simulink model "TurbochargerFullMap"  (R2014b)
settings: Solver=ode45  StartTime=0.0  StopTime=10.0  RelTol=1e-3
undefined symbols (not defined in the file or in its folder): eng
settings Model: Creator=yum  LastModifiedBy=yum

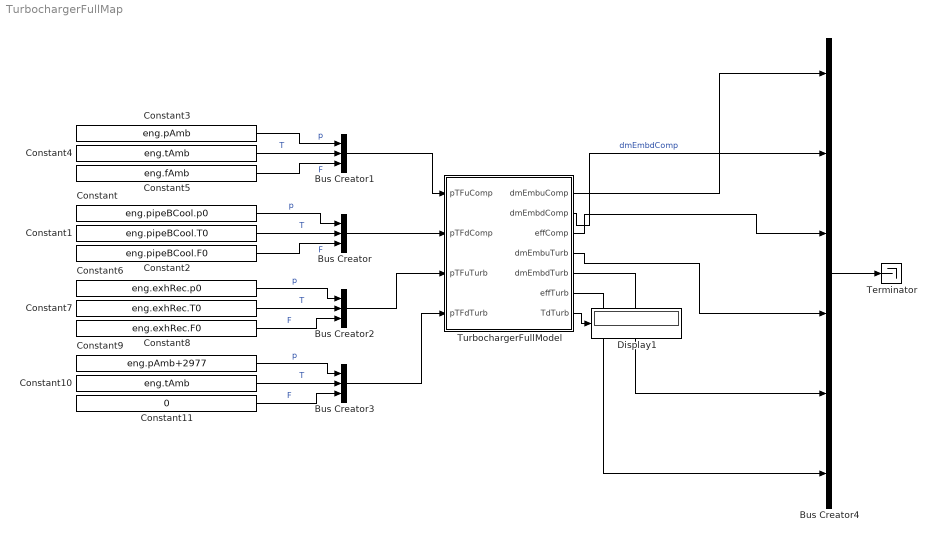
== system TurbochargerFullMap ==
  Bus Creator{,1..3} (4 alike) : BusCreator  Inputs=3
  Bus Creator4 : BusCreator  Inputs=6
  Constant : Constant  Value=eng.pipeBCool.p0
  Constant1 : Constant  Value=eng.pipeBCool.T0
  Constant10 : Constant  Value=eng.tAmb
  Constant11 : Constant  Value=0
  Constant2 : Constant  Value=eng.pipeBCool.F0
  Constant3 : Constant  Value=eng.pAmb
  Constant4 : Constant  Value=eng.tAmb
  Constant5 : Constant  Value=eng.fAmb
  Constant6 : Constant  Value=eng.exhRec.p0
  Constant7 : Constant  Value=eng.exhRec.T0
  Constant8 : Constant  Value=eng.exhRec.F0
  Constant9 : Constant  Value=eng.pAmb+2977
  Display1 : Display
  Terminator : Terminator
  TurbochargerFullModel : Subsystem  mask{turbo=eng.turbo}
      mask prompts: turbo "Turbocharger parameters"
  wires:
  Bus Creator/1 -> TurbochargerFullModel/2(pTFdComp)
  Constant/1 -> Bus Creator/1  "p"
  Constant1/1 -> Bus Creator/2  "T"
  Constant2/1 -> Bus Creator/3  "F"
  Constant4/1 -> Bus Creator1/2  "T"
  Constant5/1 -> Bus Creator1/3  "F"
  Constant3/1 -> Bus Creator1/1  "p"
  Bus Creator1/1 -> TurbochargerFullModel/1(pTFuComp)
  Constant6/1 -> Bus Creator2/1  "p"
  Constant7/1 -> Bus Creator2/2  "T"
  Constant8/1 -> Bus Creator2/3  "F"
  Bus Creator2/1 -> TurbochargerFullModel/3(pTFuTurb)
  Constant9/1 -> Bus Creator3/1  "p"
  Constant10/1 -> Bus Creator3/2  "T"
  Constant11/1 -> Bus Creator3/3  "F"
  Bus Creator3/1 -> TurbochargerFullModel/4(pTFdTurb)
  Bus Creator4/1 -> Terminator/1
  TurbochargerFullModel/3(effComp) -> Bus Creator4/3
  TurbochargerFullModel/4(dmEmbuTurb) -> Bus Creator4/4
  TurbochargerFullModel/2(dmEmbdComp) -> Bus Creator4/2  "dmEmbdComp"
  TurbochargerFullModel/5(dmEmbdTurb) -> Bus Creator4/5
  TurbochargerFullModel/1(dmEmbuComp) -> Bus Creator4/1
  TurbochargerFullModel/6(effTurb) -> Bus Creator4/6
  TurbochargerFullModel/7(TdTurb) -> Display1/1

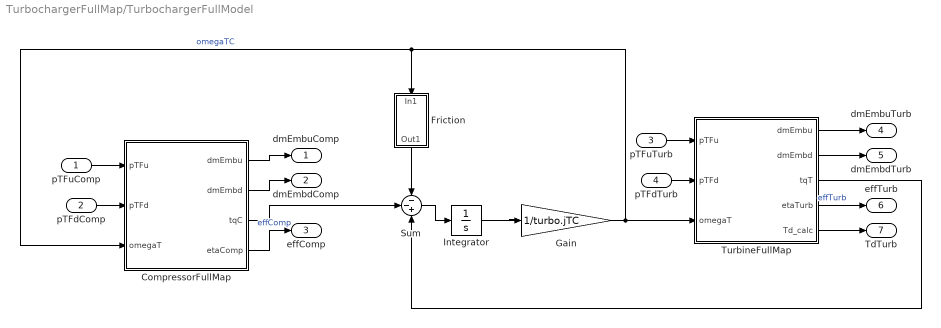
== system TurbochargerFullMap/TurbochargerFullModel ==
  pTFuComp : Inport
  pTFdComp : Inport  Port=2
  pTFuTurb : Inport  Port=3
  pTFdTurb : Inport  Port=4
  CompressorFullMap : Subsystem  mask{comp=turbo.comp}
      mask prompts: comp "Compressor Parameters"
  Friction : Subsystem
  Gain : Gain  Gain=1/turbo.jTC
  Integrator : Integrator  InitialCondition=turbo.jTC*1200
  Sum : Sum  Inputs=--+
  TurbineFullMap : Subsystem  mask{turb=turbo.turb}
      mask prompts: turb "Turbine parameters"
  dmEmbuComp : Outport
  dmEmbdComp : Outport  Port=2
  effComp : Outport  Port=3
  dmEmbuTurb : Outport  Port=4
  dmEmbdTurb : Outport  Port=5
  effTurb : Outport  Port=6
  TdTurb : Outport  Port=7
  wires:
  Integrator/1 -> Gain/1
  TurbineFullMap/3(tqT) -> Sum/3
  Sum/1 -> Integrator/1
  TurbineFullMap/4(etaTurb) -> effTurb/1  "effTurb"
  Gain/1 -> TurbineFullMap/3(omegaT), CompressorFullMap/3(omegaT), Friction/1(In1)  "omegaTC"
  pTFdTurb/1 -> TurbineFullMap/2(pTFd)
  CompressorFullMap/3(tqC) -> Sum/2
  TurbineFullMap/2(dmEmbd) -> dmEmbdTurb/1
  pTFuComp/1 -> CompressorFullMap/1(pTFu)
  CompressorFullMap/1(dmEmbu) -> dmEmbuComp/1
  pTFuTurb/1 -> TurbineFullMap/1(pTFu)
  CompressorFullMap/2(dmEmbd) -> dmEmbdComp/1
  CompressorFullMap/4(etaComp) -> effComp/1  "effComp"
  pTFdComp/1 -> CompressorFullMap/2(pTFd)
  TurbineFullMap/1(dmEmbu) -> dmEmbuTurb/1
  Friction/1(Out1) -> Sum/1
  TurbineFullMap/5(Td_calc) -> TdTurb/1

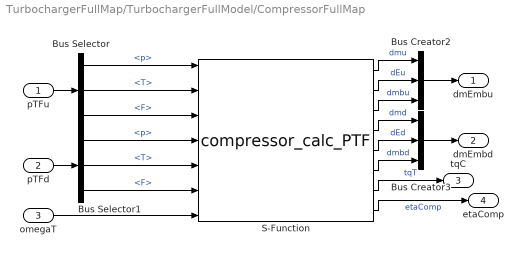
== system TurbochargerFullMap/TurbochargerFullModel/CompressorFullMap ==
  pTFu : Inport
  pTFd : Inport  Port=2
  omegaT : Inport  Port=3
  Bus Creator2 : BusCreator  Inputs=3
  Bus Creator3 : BusCreator  Inputs=3
  Bus Selector : BusSelector  OutputSignals=p,T,F
  Bus Selector1 : BusSelector  OutputSignals=p,T,F
  S-Function : S-Function  FunctionName=compressor_calc_PTF  Parameters=eng.fs,comp.flowMap,comp.effMap,comp.prRep,comp.n298Rep,int32(comp.npr),int32(comp.nsp)  EnableBusSupport=off
  dmEmbu : Outport
  dmEmbd : Outport  Port=2
  tqC : Outport  Port=3
  etaComp : Outport  Port=4
  wires:
  S-Function/7 -> tqC/1  "tqT"
  Bus Selector/1 -> S-Function/1  "<p>"
  S-Function/5 -> Bus Creator3/2  "dEd"
  omegaT/1 -> S-Function/7
  pTFu/1 -> Bus Selector/1
  pTFd/1 -> Bus Selector1/1
  Bus Selector1/2 -> S-Function/5  "<T>"
  S-Function/2 -> Bus Creator2/2  "dEu"
  Bus Creator3/1 -> dmEmbd/1
  Bus Selector1/1 -> S-Function/4  "<p>"
  Bus Selector/3 -> S-Function/3  "<F>"
  Bus Selector/2 -> S-Function/2  "<T>"
  S-Function/6 -> Bus Creator3/3  "dmbd"
  S-Function/1 -> Bus Creator2/1  "dmu"
  Bus Selector1/3 -> S-Function/6  "<F>"
  S-Function/3 -> Bus Creator2/3  "dmbu"
  S-Function/4 -> Bus Creator3/1  "dmd"
  S-Function/8 -> etaComp/1  "etaComp"
  Bus Creator2/1 -> dmEmbu/1

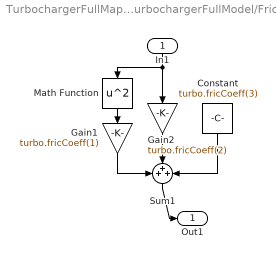
== system TurbochargerFullMap/TurbochargerFullModel/Friction ==
  In1 : Inport
  Constant : Constant  Value=turbo.fricCoeff(3)
  Gain1 : Gain  Gain=turbo.fricCoeff(1)
  Gain2 : Gain  Gain=turbo.fricCoeff(2)
  Math Function : Math  Operator=square  SaturateOnIntegerOverflow=on
  Sum1 : Sum  Inputs=+++
  Out1 : Outport
  wires:
  Sum1/1 -> Out1/1
  In1/1 -> Math Function/1, Gain2/1
  Math Function/1 -> Gain1/1
  Gain2/1 -> Sum1/2
  Gain1/1 -> Sum1/1
  Constant/1 -> Sum1/3

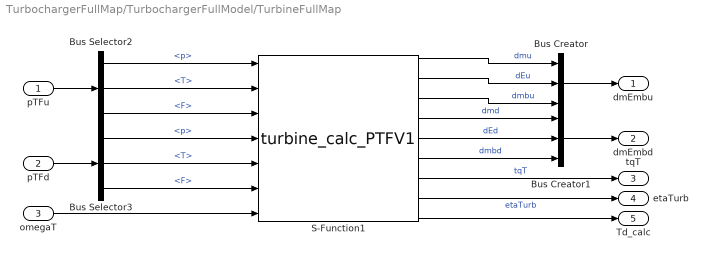
== system TurbochargerFullMap/TurbochargerFullModel/TurbineFullMap ==
  pTFu : Inport
  pTFd : Inport  Port=2
  omegaT : Inport  Port=3
  Bus Creator : BusCreator  Inputs=3
  Bus Creator1 : BusCreator  Inputs=3
  Bus Selector2 : BusSelector  OutputSignals=p,T,F
  Bus Selector3 : BusSelector  OutputSignals=p,T,F
  S-Function1 : S-Function  FunctionName=turbine_calc_PTFV1  Parameters=eng.fs,turb.flowMap,turb.effMap,turb.prRep,turb.n298Rep,int32(turb.npr),int32(turb.nsp)  EnableBusSupport=off
  dmEmbu : Outport
  dmEmbd : Outport  Port=2
  tqT : Outport  Port=3
  etaTurb : Outport  Port=4
  Td_calc : Outport  Port=5
  wires:
  Bus Selector2/2 -> S-Function1/2  "<T>"
  Bus Selector3/2 -> S-Function1/5  "<T>"
  S-Function1/3 -> Bus Creator/3  "dmbu"
  Bus Selector2/3 -> S-Function1/3  "<F>"
  S-Function1/6 -> Bus Creator1/3  "dmbd"
  omegaT/1 -> S-Function1/7
  S-Function1/8 -> etaTurb/1  "etaTurb"
  S-Function1/1 -> Bus Creator/1  "dmu"
  pTFu/1 -> Bus Selector2/1
  Bus Selector2/1 -> S-Function1/1  "<p>"
  pTFd/1 -> Bus Selector3/1
  Bus Selector3/1 -> S-Function1/4  "<p>"
  S-Function1/5 -> Bus Creator1/2  "dEd"
  S-Function1/7 -> tqT/1  "tqT"
  Bus Selector3/3 -> S-Function1/6  "<F>"
  S-Function1/2 -> Bus Creator/2  "dEu"
  S-Function1/4 -> Bus Creator1/1  "dmd"
  Bus Creator/1 -> dmEmbu/1
  Bus Creator1/1 -> dmEmbd/1
  S-Function1/9 -> Td_calc/1
